simulink model "FSAC2021_V1"  (R2014a)
settings: Solver=FixedStepDiscrete  StartTime=0.0  StopTime=inf  FixedStep=0.0005  RelTol=1e-3
model workspace (MAT data in the model file):
  MCOS : class17 (value not decoded)
  MCOS : class17 (value not decoded)
  MCOS : class17 (value not decoded)
  MCOS : class17 (value not decoded)
  MCOS : class17 (value not decoded)
  MCOS : class17 (value not decoded)
  MCOS : class17 (value not decoded)
  MCOS : class17 (value not decoded)
  MCOS : class17 (value not decoded)
  MCOS : class17 (value not decoded)
  MCOS : class17 (value not decoded)
  MCOS : class17 (value not decoded)
  MCOS : class17 (value not decoded)
  MCOS : class17 (value not decoded)
  MCOS : class17 (value not decoded)
  MCOS : class17 (value not decoded)
  MCOS : class17 (value not decoded)
  MCOS : class17 (value not decoded)
  MCOS : class17 (value not decoded)
  BUZZER_START = 1
  MCOS : class17 (value not decoded)
  MCOS : class17 (value not decoded)
  MCOS : class17 (value not decoded)
  MCOS : class17 (value not decoded)
  MCOS : class17 (value not decoded)
  MCOS : class17 (value not decoded)
  MCOS : class17 (value not decoded)
  MCOS : class17 (value not decoded)
  MCOS : class17 (value not decoded)
  MCOS : class17 (value not decoded)
  MCOS : class17 (value not decoded)
  MCOS : class17 (value not decoded)
  MCOS : class17 (value not decoded)
  MCOS : class17 (value not decoded)
  MCOS : class17 (value not decoded)
  MCOS : class17 (value not decoded)
  MCOS : class17 (value not decoded)
  MCOS : class17 (value not decoded)
  MCOS : class17 (value not decoded)
  MCOS : class17 (value not decoded)
  MCOS : class17 (value not decoded)
  MCOS : class17 (value not decoded)
  MCOS : class17 (value not decoded)
  MCOS : class17 (value not decoded)
  MCOS : class17 (value not decoded)
  MCOS : class17 (value not decoded)
  MCOS : class17 (value not decoded)
  MCOS : class17 (value not decoded)
  MCOS : class17 (value not decoded)
  MCOS : class17 (value not decoded)
  MCOS : class17 (value not decoded)
  MCOS : class17 (value not decoded)
  MCOS : class17 (value not decoded)
  MCOS : class17 (value not decoded)
  MCOS : class17 (value not decoded)
  MCOS : class17 (value not decoded)
  MCOS : class17 (value not decoded)
  MCOS : class17 (value not decoded)
  Brake = 11
  MCOS : class17 (value not decoded)
  MCOS : class17 (value not decoded)
  MCOS : class17 (value not decoded)
  MCOS : class17 (value not decoded)
  MCOS : class17 (value not decoded)
  MCOS : class17 (value not decoded)
  MCOS : class17 (value not decoded)
  MCOS : class17 (value not decoded)
  Sensor_Acc_b = 101.85
  Sensor_Acc_k = -0.0185
  Str_Sen_Orig_Angle = -341
  MCOS : class17 (value not decoded)
  Tire_D = 0.47
  T = 0.05
libraries: simulink x189, ec55xxlib x135
(part 8 of 9)

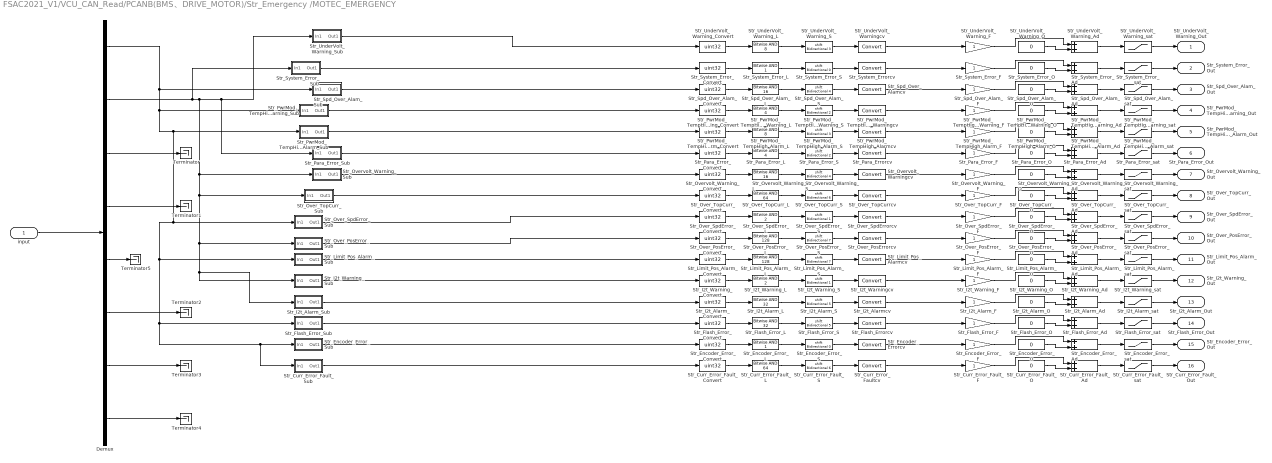
== system FSAC2021_V1/VCU_CAN_Read/PCANB(BMS、DRIVE_MOTOR)/Str_Emergency /MOTEC_EMERGENCY ==
  input : Inport
  Demux : Demux  Outputs=8
  Str_Curr_Error_Fault_Ad : Sum
  Str_Curr_Error_Fault_Convert : DataTypeConversion  OutDataTypeStr=uint32
  Str_Curr_Error_Fault_F : Gain
  Str_Curr_Error_Fault_L : simulink/Logic and Bit Operations/Bitwise Operator  logicop=AND  UseBitMask=on  BitMask=64  BitMaskRealWorld=Stored Integer
  Str_Curr_Error_Fault_O : Constant  Value=0  OutDataTypeStr=single
  Str_Curr_Error_Fault_S : ArithShift  BitShiftNumber=6
  Str_Curr_Error_Fault_Sub : Subsystem
  Str_Curr_Error_Fault_sat : Saturate  UpperLimit=1  LowerLimit=0
  Str_Curr_Error_Faultcv : DataTypeConversion
  Str_Encoder_Error_Ad : Sum
  Str_Encoder_Error_Convert : DataTypeConversion  OutDataTypeStr=uint32
  Str_Encoder_Error_F : Gain
  Str_Encoder_Error_L : simulink/Logic and Bit Operations/Bitwise Operator  logicop=AND  UseBitMask=on  BitMask=1  BitMaskRealWorld=Stored Integer
  Str_Encoder_Error_O : Constant  Value=0  OutDataTypeStr=single
  Str_Encoder_Error_S : ArithShift
  Str_Encoder_Error_Sub : Subsystem
  Str_Encoder_Error_sat : Saturate  UpperLimit=1  LowerLimit=0
  Str_Encoder_Errorcv : DataTypeConversion
  Str_Flash_Error_Ad : Sum
  Str_Flash_Error_Convert : DataTypeConversion  OutDataTypeStr=uint32
  Str_Flash_Error_F : Gain
  Str_Flash_Error_L : simulink/Logic and Bit Operations/Bitwise Operator  logicop=AND  UseBitMask=on  BitMask=32  BitMaskRealWorld=Stored Integer
  Str_Flash_Error_O : Constant  Value=0  OutDataTypeStr=single
  Str_Flash_Error_S : ArithShift  BitShiftNumber=5
  Str_Flash_Error_Sub : Subsystem
  Str_Flash_Error_sat : Saturate  UpperLimit=1  LowerLimit=0
  Str_Flash_Errorcv : DataTypeConversion
  Str_I2t_Alarm_Ad : Sum
  Str_I2t_Alarm_Convert : DataTypeConversion  OutDataTypeStr=uint32
  Str_I2t_Alarm_F : Gain
  Str_I2t_Alarm_L : simulink/Logic and Bit Operations/Bitwise Operator  logicop=AND  UseBitMask=on  BitMask=32  BitMaskRealWorld=Stored Integer
  Str_I2t_Alarm_O : Constant  Value=0  OutDataTypeStr=single
  Str_I2t_Alarm_S : ArithShift  BitShiftNumber=5
  Str_I2t_Alarm_Sub : Subsystem
  Str_I2t_Alarm_sat : Saturate  UpperLimit=1  LowerLimit=0
  Str_I2t_Alarmcv : DataTypeConversion
  Str_I2t_Warning_Ad : Sum
  Str_I2t_Warning_Convert : DataTypeConversion  OutDataTypeStr=uint32
  Str_I2t_Warning_F : Gain
  Str_I2t_Warning_L : simulink/Logic and Bit Operations/Bitwise Operator  logicop=AND  UseBitMask=on  BitMask=2  BitMaskRealWorld=Stored Integer
  Str_I2t_Warning_O : Constant  Value=0  OutDataTypeStr=single
  Str_I2t_Warning_S : ArithShift  BitShiftNumber=1
  Str_I2t_Warning_Sub : Subsystem
  Str_I2t_Warning_sat : Saturate  UpperLimit=1  LowerLimit=0
  Str_I2t_Warningcv : DataTypeConversion
  Str_Limit_Pos_Alarm_Ad : Sum
  Str_Limit_Pos_Alarm_Convert : DataTypeConversion  OutDataTypeStr=uint32
  Str_Limit_Pos_Alarm_F : Gain
  Str_Limit_Pos_Alarm_L : simulink/Logic and Bit Operations/Bitwise Operator  logicop=AND  UseBitMask=on  BitMask=128  BitMaskRealWorld=Stored Integer
  Str_Limit_Pos_Alarm_O : Constant  Value=0  OutDataTypeStr=single
  Str_Limit_Pos_Alarm_S : ArithShift  BitShiftNumber=7
  Str_Limit_Pos_Alarm_Sub : Subsystem
  Str_Limit_Pos_Alarm_sat : Saturate  UpperLimit=1  LowerLimit=0
  Str_Limit_Pos_Alarmcv : DataTypeConversion
  Str_Over_PosError_Ad : Sum
  Str_Over_PosError_Convert : DataTypeConversion  OutDataTypeStr=uint32
  Str_Over_PosError_F : Gain
  Str_Over_PosError_L : simulink/Logic and Bit Operations/Bitwise Operator  logicop=AND  UseBitMask=on  BitMask=128  BitMaskRealWorld=Stored Integer
  Str_Over_PosError_O : Constant  Value=0  OutDataTypeStr=single
  Str_Over_PosError_S : ArithShift  BitShiftNumber=7
  Str_Over_PosError_Sub : Subsystem
  Str_Over_PosError_sat : Saturate  UpperLimit=1  LowerLimit=0
  Str_Over_PosErrorcv : DataTypeConversion
  Str_Over_SpdError_Ad : Sum
  Str_Over_SpdError_Convert : DataTypeConversion  OutDataTypeStr=uint32
  Str_Over_SpdError_F : Gain
  Str_Over_SpdError_L : simulink/Logic and Bit Operations/Bitwise Operator  logicop=AND  UseBitMask=on  BitMask=2  BitMaskRealWorld=Stored Integer
  Str_Over_SpdError_O : Constant  Value=0  OutDataTypeStr=single
  Str_Over_SpdError_S : ArithShift  BitShiftNumber=1
  Str_Over_SpdError_Sub : Subsystem
  Str_Over_SpdError_sat : Saturate  UpperLimit=1  LowerLimit=0
  Str_Over_SpdErrorcv : DataTypeConversion
  Str_Over_TopCurr_Ad : Sum
  Str_Over_TopCurr_Convert : DataTypeConversion  OutDataTypeStr=uint32
  Str_Over_TopCurr_F : Gain
  Str_Over_TopCurr_L : simulink/Logic and Bit Operations/Bitwise Operator  logicop=AND  UseBitMask=on  BitMask=64  BitMaskRealWorld=Stored Integer
  Str_Over_TopCurr_O : Constant  Value=0  OutDataTypeStr=single
  Str_Over_TopCurr_S : ArithShift  BitShiftNumber=6
  Str_Over_TopCurr_Sub : Subsystem
  Str_Over_TopCurr_sat : Saturate  UpperLimit=1  LowerLimit=0
  Str_Over_TopCurrcv : DataTypeConversion
  Str_Overvolt_Warning_Ad : Sum
  Str_Overvolt_Warning_Convert : DataTypeConversion  OutDataTypeStr=uint32
  Str_Overvolt_Warning_F : Gain
  Str_Overvolt_Warning_L : simulink/Logic and Bit Operations/Bitwise Operator  logicop=AND  UseBitMask=on  BitMask=16  BitMaskRealWorld=Stored Integer
  Str_Overvolt_Warning_O : Constant  Value=0  OutDataTypeStr=single
  Str_Overvolt_Warning_S : ArithShift  BitShiftNumber=4
  Str_Overvolt_Warning_Sub : Subsystem
  Str_Overvolt_Warning_sat : Saturate  UpperLimit=1  LowerLimit=0
  Str_Overvolt_Warningcv : DataTypeConversion
  Str_Para_Error_Ad : Sum
  Str_Para_Error_Convert : DataTypeConversion  OutDataTypeStr=uint32
  Str_Para_Error_F : Gain
  Str_Para_Error_L : simulink/Logic and Bit Operations/Bitwise Operator  logicop=AND  UseBitMask=on  BitMask=4  BitMaskRealWorld=Stored Integer
  Str_Para_Error_O : Constant  Value=0  OutDataTypeStr=single
  Str_Para_Error_S : ArithShift  BitShiftNumber=2
  Str_Para_Error_Sub : Subsystem
  Str_Para_Error_sat : Saturate  UpperLimit=1  LowerLimit=0
  Str_Para_Errorcv : DataTypeConversion
  Str_PwrMod_TempHigh_Alarm_Ad : Sum
  Str_PwrMod_TempHigh_Alarm_Convert : DataTypeConversion  OutDataTypeStr=uint32
  Str_PwrMod_TempHigh_Alarm_F : Gain
  Str_PwrMod_TempHigh_Alarm_L : simulink/Logic and Bit Operations/Bitwise Operator  logicop=AND  UseBitMask=on  BitMask=8  BitMaskRealWorld=Stored Integer
  Str_PwrMod_TempHigh_Alarm_O : Constant  Value=0  OutDataTypeStr=single
  Str_PwrMod_TempHigh_Alarm_S : ArithShift  BitShiftNumber=3
  Str_PwrMod_TempHigh_Alarm_Sub : Subsystem
  Str_PwrMod_TempHigh_Alarm_sat : Saturate  UpperLimit=1  LowerLimit=0
  Str_PwrMod_TempHigh_Alarmcv : DataTypeConversion
  Str_PwrMod_TempHigh_Warning_Ad : Sum
  Str_PwrMod_TempHigh_Warning_Convert : DataTypeConversion  OutDataTypeStr=uint32
  Str_PwrMod_TempHigh_Warning_F : Gain
  Str_PwrMod_TempHigh_Warning_L : simulink/Logic and Bit Operations/Bitwise Operator  logicop=AND  UseBitMask=on  BitMask=4  BitMaskRealWorld=Stored Integer
  Str_PwrMod_TempHigh_Warning_O : Constant  Value=0  OutDataTypeStr=single
  Str_PwrMod_TempHigh_Warning_S : ArithShift  BitShiftNumber=2
  Str_PwrMod_TempHigh_Warning_Sub : Subsystem
  Str_PwrMod_TempHigh_Warning_sat : Saturate  UpperLimit=1  LowerLimit=0
  Str_PwrMod_TempHigh_Warningcv : DataTypeConversion
  Str_Spd_Over_Alam_Ad : Sum
  Str_Spd_Over_Alam_Convert : DataTypeConversion  OutDataTypeStr=uint32
  Str_Spd_Over_Alam_F : Gain
  Str_Spd_Over_Alam_L : simulink/Logic and Bit Operations/Bitwise Operator  logicop=AND  UseBitMask=on  BitMask=16  BitMaskRealWorld=Stored Integer
  Str_Spd_Over_Alam_O : Constant  Value=0  OutDataTypeStr=single
  Str_Spd_Over_Alam_S : ArithShift  BitShiftNumber=4
  Str_Spd_Over_Alam_Sub : Subsystem
  Str_Spd_Over_Alam_sat : Saturate  UpperLimit=1  LowerLimit=0
  Str_Spd_Over_Alamcv : DataTypeConversion
  Str_System_Error_Ad : Sum
  Str_System_Error_Convert : DataTypeConversion  OutDataTypeStr=uint32
  Str_System_Error_F : Gain
  Str_System_Error_L : simulink/Logic and Bit Operations/Bitwise Operator  logicop=AND  UseBitMask=on  BitMask=1  BitMaskRealWorld=Stored Integer
  Str_System_Error_O : Constant  Value=0  OutDataTypeStr=single
  Str_System_Error_S : ArithShift
  Str_System_Error_Sub : Subsystem
  Str_System_Error_sat : Saturate  UpperLimit=1  LowerLimit=0
  Str_System_Errorcv : DataTypeConversion
  Str_UnderVolt_Warning_Ad : Sum
  Str_UnderVolt_Warning_Convert : DataTypeConversion  OutDataTypeStr=uint32
  Str_UnderVolt_Warning_F : Gain
  Str_UnderVolt_Warning_L : simulink/Logic and Bit Operations/Bitwise Operator  logicop=AND  UseBitMask=on  BitMask=8  BitMaskRealWorld=Stored Integer
  Str_UnderVolt_Warning_O : Constant  Value=0  OutDataTypeStr=single
  Str_UnderVolt_Warning_S : ArithShift  BitShiftNumber=3
  Str_UnderVolt_Warning_Sub : Subsystem
  Str_UnderVolt_Warning_sat : Saturate  UpperLimit=1  LowerLimit=0
  Str_UnderVolt_Warningcv : DataTypeConversion
  Terminator{,1..5} (6 alike) : Terminator
  Str_UnderVolt_Warning_Out : Outport
  Str_System_Error_Out : Outport  Port=2
  Str_Spd_Over_Alam_Out : Outport  Port=3
  Str_PwrMod_TempHigh_Warning_Out : Outport  Port=4
  Str_PwrMod_TempHigh_Alarm_Out : Outport  Port=5
  Str_Para_Error_Out : Outport  Port=6
  Str_Overvolt_Warning_Out : Outport  Port=7
  Str_Over_TopCurr_Out : Outport  Port=8
  Str_Over_SpdError_Out : Outport  Port=9
  Str_Over_PosError_Out : Outport  Port=10
  Str_Limit_Pos_Alarm_Out : Outport  Port=11
  Str_I2t_Warning_Out : Outport  Port=12
  Str_I2t_Alarm_Out : Outport  Port=13
  Str_Flash_Error_Out : Outport  Port=14
  Str_Encoder_Error_Out : Outport  Port=15
  Str_Curr_Error_Fault_Out : Outport  Port=16
  wires:
  Str_UnderVolt_Warning_F/1 -> Str_UnderVolt_Warning_Ad/1
  Str_UnderVolt_Warning_O/1 -> Str_UnderVolt_Warning_Ad/2
  Str_UnderVolt_Warning_Ad/1 -> Str_UnderVolt_Warning_sat/1
  Str_UnderVolt_Warning_sat/1 -> Str_UnderVolt_Warning_Out/1
  Demux/2 -> Str_Para_Error_Sub/1(In1), Str_UnderVolt_Warning_Sub/1(In1), Str_I2t_Warning_Sub/1(In1), Str_I2t_Alarm_Sub/1(In1), Str_Over_PosError_Sub/1(In1), Str_Over_TopCurr_Sub/1(In1), Str_Overvolt_Warning_Sub/1(In1), Str_System_Error_Sub/1(In1)
  Str_UnderVolt_Warning_Sub/1(Out1) -> Str_UnderVolt_Warning_Convert/1
  Str_UnderVolt_Warning_Convert/1 -> Str_UnderVolt_Warning_L/1
  Str_UnderVolt_Warning_L/1 -> Str_UnderVolt_Warning_S/1
  Str_UnderVolt_Warning_S/1 -> Str_UnderVolt_Warningcv/1
  Str_UnderVolt_Warningcv/1 -> Str_UnderVolt_Warning_F/1
  Str_System_Error_F/1 -> Str_System_Error_Ad/1
  Str_System_Error_O/1 -> Str_System_Error_Ad/2
  Str_System_Error_Ad/1 -> Str_System_Error_sat/1
  Str_System_Error_sat/1 -> Str_System_Error_Out/1
  Str_System_Error_Sub/1(Out1) -> Str_System_Error_Convert/1
  Str_System_Error_Convert/1 -> Str_System_Error_L/1
  Str_System_Error_L/1 -> Str_System_Error_S/1
  Str_System_Error_S/1 -> Str_System_Errorcv/1
  Str_System_Errorcv/1 -> Str_System_Error_F/1
  Str_Spd_Over_Alam_F/1 -> Str_Spd_Over_Alam_Ad/1
  Str_Spd_Over_Alam_O/1 -> Str_Spd_Over_Alam_Ad/2
  Str_Spd_Over_Alam_Ad/1 -> Str_Spd_Over_Alam_sat/1
  Str_Spd_Over_Alam_sat/1 -> Str_Spd_Over_Alam_Out/1
  Demux/1 -> Str_Encoder_Error_Sub/1(In1), Str_Curr_Error_Fault_Sub/1(In1), Str_Flash_Error_Sub/1(In1), Str_Limit_Pos_Alarm_Sub/1(In1), Str_Over_SpdError_Sub/1(In1), Str_PwrMod_TempHigh_Alarm_Sub/1(In1), Str_PwrMod_TempHigh_Warning_Sub/1(In1), Str_Spd_Over_Alam_Sub/1(In1)
  Str_Spd_Over_Alam_Sub/1(Out1) -> Str_Spd_Over_Alam_Convert/1
  Str_Spd_Over_Alam_Convert/1 -> Str_Spd_Over_Alam_L/1
  Str_Spd_Over_Alam_L/1 -> Str_Spd_Over_Alam_S/1
  Str_Spd_Over_Alam_S/1 -> Str_Spd_Over_Alamcv/1
  Str_Spd_Over_Alamcv/1 -> Str_Spd_Over_Alam_F/1
  Str_PwrMod_TempHigh_Warning_F/1 -> Str_PwrMod_TempHigh_Warning_Ad/1
  Str_PwrMod_TempHigh_Warning_O/1 -> Str_PwrMod_TempHigh_Warning_Ad/2
  Str_PwrMod_TempHigh_Warning_Ad/1 -> Str_PwrMod_TempHigh_Warning_sat/1
  Str_PwrMod_TempHigh_Warning_sat/1 -> Str_PwrMod_TempHigh_Warning_Out/1
  Str_PwrMod_TempHigh_Warning_Sub/1(Out1) -> Str_PwrMod_TempHigh_Warning_Convert/1
  Str_PwrMod_TempHigh_Warning_Convert/1 -> Str_PwrMod_TempHigh_Warning_L/1
  Str_PwrMod_TempHigh_Warning_L/1 -> Str_PwrMod_TempHigh_Warning_S/1
  Str_PwrMod_TempHigh_Warning_S/1 -> Str_PwrMod_TempHigh_Warningcv/1
  Str_PwrMod_TempHigh_Warningcv/1 -> Str_PwrMod_TempHigh_Warning_F/1
  Str_PwrMod_TempHigh_Alarm_F/1 -> Str_PwrMod_TempHigh_Alarm_Ad/1
  Str_PwrMod_TempHigh_Alarm_O/1 -> Str_PwrMod_TempHigh_Alarm_Ad/2
  Str_PwrMod_TempHigh_Alarm_Ad/1 -> Str_PwrMod_TempHigh_Alarm_sat/1
  Str_PwrMod_TempHigh_Alarm_sat/1 -> Str_PwrMod_TempHigh_Alarm_Out/1
  Str_PwrMod_TempHigh_Alarm_Sub/1(Out1) -> Str_PwrMod_TempHigh_Alarm_Convert/1
  Str_PwrMod_TempHigh_Alarm_Convert/1 -> Str_PwrMod_TempHigh_Alarm_L/1
  Str_PwrMod_TempHigh_Alarm_L/1 -> Str_PwrMod_TempHigh_Alarm_S/1
  Str_PwrMod_TempHigh_Alarm_S/1 -> Str_PwrMod_TempHigh_Alarmcv/1
  Str_PwrMod_TempHigh_Alarmcv/1 -> Str_PwrMod_TempHigh_Alarm_F/1
  Str_Para_Error_F/1 -> Str_Para_Error_Ad/1
  Str_Para_Error_O/1 -> Str_Para_Error_Ad/2
  Str_Para_Error_Ad/1 -> Str_Para_Error_sat/1
  Str_Para_Error_sat/1 -> Str_Para_Error_Out/1
  Str_Para_Error_Sub/1(Out1) -> Str_Para_Error_Convert/1
  Str_Para_Error_Convert/1 -> Str_Para_Error_L/1
  Str_Para_Error_L/1 -> Str_Para_Error_S/1
  Str_Para_Error_S/1 -> Str_Para_Errorcv/1
  Str_Para_Errorcv/1 -> Str_Para_Error_F/1
  Str_Overvolt_Warning_F/1 -> Str_Overvolt_Warning_Ad/1
  Str_Overvolt_Warning_O/1 -> Str_Overvolt_Warning_Ad/2
  Str_Overvolt_Warning_Ad/1 -> Str_Overvolt_Warning_sat/1
  Str_Overvolt_Warning_sat/1 -> Str_Overvolt_Warning_Out/1
  Str_Overvolt_Warning_Sub/1(Out1) -> Str_Overvolt_Warning_Convert/1
  Str_Overvolt_Warning_Convert/1 -> Str_Overvolt_Warning_L/1
  Str_Overvolt_Warning_L/1 -> Str_Overvolt_Warning_S/1
  Str_Overvolt_Warning_S/1 -> Str_Overvolt_Warningcv/1
  Str_Overvolt_Warningcv/1 -> Str_Overvolt_Warning_F/1
  Str_Over_TopCurr_F/1 -> Str_Over_TopCurr_Ad/1
  Str_Over_TopCurr_O/1 -> Str_Over_TopCurr_Ad/2
  Str_Over_TopCurr_Ad/1 -> Str_Over_TopCurr_sat/1
  Str_Over_TopCurr_sat/1 -> Str_Over_TopCurr_Out/1
  Str_Over_TopCurr_Sub/1(Out1) -> Str_Over_TopCurr_Convert/1
  Str_Over_TopCurr_Convert/1 -> Str_Over_TopCurr_L/1
  Str_Over_TopCurr_L/1 -> Str_Over_TopCurr_S/1
  Str_Over_TopCurr_S/1 -> Str_Over_TopCurrcv/1
  Str_Over_TopCurrcv/1 -> Str_Over_TopCurr_F/1
  Str_Over_SpdError_F/1 -> Str_Over_SpdError_Ad/1
  Str_Over_SpdError_O/1 -> Str_Over_SpdError_Ad/2
  Str_Over_SpdError_Ad/1 -> Str_Over_SpdError_sat/1
  Str_Over_SpdError_sat/1 -> Str_Over_SpdError_Out/1
  Str_Over_SpdError_Sub/1(Out1) -> Str_Over_SpdError_Convert/1
  Str_Over_SpdError_Convert/1 -> Str_Over_SpdError_L/1
  Str_Over_SpdError_L/1 -> Str_Over_SpdError_S/1
  Str_Over_SpdError_S/1 -> Str_Over_SpdErrorcv/1
  Str_Over_SpdErrorcv/1 -> Str_Over_SpdError_F/1
  Str_Over_PosError_F/1 -> Str_Over_PosError_Ad/1
  Str_Over_PosError_O/1 -> Str_Over_PosError_Ad/2
  Str_Over_PosError_Ad/1 -> Str_Over_PosError_sat/1
  Str_Over_PosError_sat/1 -> Str_Over_PosError_Out/1
  Str_Over_PosError_Sub/1(Out1) -> Str_Over_PosError_Convert/1
  Str_Over_PosError_Convert/1 -> Str_Over_PosError_L/1
  Str_Over_PosError_L/1 -> Str_Over_PosError_S/1
  Str_Over_PosError_S/1 -> Str_Over_PosErrorcv/1
  Str_Over_PosErrorcv/1 -> Str_Over_PosError_F/1
  Str_Limit_Pos_Alarm_F/1 -> Str_Limit_Pos_Alarm_Ad/1
  Str_Limit_Pos_Alarm_O/1 -> Str_Limit_Pos_Alarm_Ad/2
  Str_Limit_Pos_Alarm_Ad/1 -> Str_Limit_Pos_Alarm_sat/1
  Str_Limit_Pos_Alarm_sat/1 -> Str_Limit_Pos_Alarm_Out/1
  Str_Limit_Pos_Alarm_Sub/1(Out1) -> Str_Limit_Pos_Alarm_Convert/1
  Str_Limit_Pos_Alarm_Convert/1 -> Str_Limit_Pos_Alarm_L/1
  Str_Limit_Pos_Alarm_L/1 -> Str_Limit_Pos_Alarm_S/1
  Str_Limit_Pos_Alarm_S/1 -> Str_Limit_Pos_Alarmcv/1
  Str_Limit_Pos_Alarmcv/1 -> Str_Limit_Pos_Alarm_F/1
  Str_I2t_Warning_F/1 -> Str_I2t_Warning_Ad/1
  Str_I2t_Warning_O/1 -> Str_I2t_Warning_Ad/2
  Str_I2t_Warning_Ad/1 -> Str_I2t_Warning_sat/1
  Str_I2t_Warning_sat/1 -> Str_I2t_Warning_Out/1
  Str_I2t_Warning_Sub/1(Out1) -> Str_I2t_Warning_Convert/1
  Str_I2t_Warning_Convert/1 -> Str_I2t_Warning_L/1
  Str_I2t_Warning_L/1 -> Str_I2t_Warning_S/1
  Str_I2t_Warning_S/1 -> Str_I2t_Warningcv/1
  Str_I2t_Warningcv/1 -> Str_I2t_Warning_F/1
  Str_I2t_Alarm_F/1 -> Str_I2t_Alarm_Ad/1
  Str_I2t_Alarm_O/1 -> Str_I2t_Alarm_Ad/2
  Str_I2t_Alarm_Ad/1 -> Str_I2t_Alarm_sat/1
  Str_I2t_Alarm_sat/1 -> Str_I2t_Alarm_Out/1
  Str_I2t_Alarm_Sub/1(Out1) -> Str_I2t_Alarm_Convert/1
  Str_I2t_Alarm_Convert/1 -> Str_I2t_Alarm_L/1
  Str_I2t_Alarm_L/1 -> Str_I2t_Alarm_S/1
  Str_I2t_Alarm_S/1 -> Str_I2t_Alarmcv/1
  Str_I2t_Alarmcv/1 -> Str_I2t_Alarm_F/1
  Str_Flash_Error_F/1 -> Str_Flash_Error_Ad/1
  Str_Flash_Error_O/1 -> Str_Flash_Error_Ad/2
  Str_Flash_Error_Ad/1 -> Str_Flash_Error_sat/1
  Str_Flash_Error_sat/1 -> Str_Flash_Error_Out/1
  Str_Flash_Error_Sub/1(Out1) -> Str_Flash_Error_Convert/1
  Str_Flash_Error_Convert/1 -> Str_Flash_Error_L/1
  Str_Flash_Error_L/1 -> Str_Flash_Error_S/1
  Str_Flash_Error_S/1 -> Str_Flash_Errorcv/1
  Str_Flash_Errorcv/1 -> Str_Flash_Error_F/1
  Str_Encoder_Error_F/1 -> Str_Encoder_Error_Ad/1
  Str_Encoder_Error_O/1 -> Str_Encoder_Error_Ad/2
  Str_Encoder_Error_Ad/1 -> Str_Encoder_Error_sat/1
  Str_Encoder_Error_sat/1 -> Str_Encoder_Error_Out/1
  Str_Encoder_Error_Sub/1(Out1) -> Str_Encoder_Error_Convert/1
  Str_Encoder_Error_Convert/1 -> Str_Encoder_Error_L/1
  Str_Encoder_Error_L/1 -> Str_Encoder_Error_S/1
  Str_Encoder_Error_S/1 -> Str_Encoder_Errorcv/1
  Str_Encoder_Errorcv/1 -> Str_Encoder_Error_F/1
  Str_Curr_Error_Fault_F/1 -> Str_Curr_Error_Fault_Ad/1
  Str_Curr_Error_Fault_O/1 -> Str_Curr_Error_Fault_Ad/2
  Str_Curr_Error_Fault_Ad/1 -> Str_Curr_Error_Fault_sat/1
  Str_Curr_Error_Fault_sat/1 -> Str_Curr_Error_Fault_Out/1
  Str_Curr_Error_Fault_Sub/1(Out1) -> Str_Curr_Error_Fault_Convert/1
  Str_Curr_Error_Fault_Convert/1 -> Str_Curr_Error_Fault_L/1
  Str_Curr_Error_Fault_L/1 -> Str_Curr_Error_Fault_S/1
  Str_Curr_Error_Fault_S/1 -> Str_Curr_Error_Faultcv/1
  Str_Curr_Error_Faultcv/1 -> Str_Curr_Error_Fault_F/1
  input/1 -> Demux/1
  Demux/3 -> Terminator/1
  Demux/4 -> Terminator1/1
  Demux/6 -> Terminator2/1
  Demux/7 -> Terminator3/1
  Demux/8 -> Terminator4/1
  Demux/5 -> Terminator5/1

== system FSAC2021_V1/VCU_CAN_Read/Subsystem/BMS_HCU_INFO /BMS_HCU_INFO ==
  input : Inport
  BatAlmLv_Ad : Sum
  BatAlmLv_Convert : DataTypeConversion  OutDataTypeStr=uint32
  BatAlmLv_F : Gain
  BatAlmLv_L : simulink/Logic and Bit Operations/Bitwise Operator  logicop=AND  UseBitMask=on  BitMask=15  BitMaskRealWorld=Stored Integer
  BatAlmLv_O : Constant  Value=0  OutDataTypeStr=single
  BatAlmLv_S : ArithShift
  BatAlmLv_Sub : Subsystem
  BatAlmLv_sat : Saturate  UpperLimit=4  LowerLimit=0
  BatAlmLvcv : DataTypeConversion
  BatCurrent_Ad : Sum
  BatCurrent_Convert : DataTypeConversion  OutDataTypeStr=uint32
  BatCurrent_F : Gain  Gain=0.1
  BatCurrent_L : simulink/Logic and Bit Operations/Bitwise Operator  logicop=AND  UseBitMask=on  BitMask=65535  BitMaskRealWorld=Stored Integer
  BatCurrent_O : Constant  Value=-1000  OutDataTypeStr=single
  BatCurrent_S : ArithShift
  BatCurrent_Sub : Subsystem
  BatCurrent_sat : Saturate  UpperLimit=1000  LowerLimit=-1000
  BatCurrentcv : DataTypeConversion
  BatCurrentinput3_Ad : Sum
  BatCurrentinput3_C : Constant  Value=256
  BatCurrentinput3_P : Product
  BatLife_Ad : Sum
  BatLife_Convert : DataTypeConversion  OutDataTypeStr=uint32
  BatLife_F : Gain
  BatLife_L : simulink/Logic and Bit Operations/Bitwise Operator  logicop=AND  UseBitMask=on  BitMask=255  BitMaskRealWorld=Stored Integer
  BatLife_O : Constant  Value=0  OutDataTypeStr=single
  BatLife_S : ArithShift
  BatLife_Sub : Subsystem
  BatLife_sat : Saturate  UpperLimit=255  LowerLimit=0
  BatLifecv : DataTypeConversion
  BatSoc_Ad : Sum
  BatSoc_Convert : DataTypeConversion  OutDataTypeStr=uint32
  BatSoc_F : Gain
  BatSoc_L : simulink/Logic and Bit Operations/Bitwise Operator  logicop=AND  UseBitMask=on  BitMask=255  BitMaskRealWorld=Stored Integer
  BatSoc_O : Constant  Value=0  OutDataTypeStr=single
  BatSoc_S : ArithShift
  BatSoc_Sub : Subsystem
  BatSoc_sat : Saturate  UpperLimit=100  LowerLimit=0
  BatSoccv : DataTypeConversion
  BatSoh_Ad : Sum
  BatSoh_Convert : DataTypeConversion  OutDataTypeStr=uint32
  BatSoh_F : Gain
  BatSoh_L : simulink/Logic and Bit Operations/Bitwise Operator  logicop=AND  UseBitMask=on  BitMask=255  BitMaskRealWorld=Stored Integer
  BatSoh_O : Constant  Value=0  OutDataTypeStr=single
  BatSoh_S : ArithShift
  BatSoh_Sub : Subsystem
  BatSoh_sat : Saturate  UpperLimit=100  LowerLimit=0
  BatSohcv : DataTypeConversion
  BatState_Ad : Sum
  BatState_Convert : DataTypeConversion  OutDataTypeStr=uint32
  BatState_F : Gain
  BatState_L : simulink/Logic and Bit Operations/Bitwise Operator  logicop=AND  UseBitMask=on  BitMask=240  BitMaskRealWorld=Stored Integer
  BatState_O : Constant  Value=0  OutDataTypeStr=single
  BatState_S : ArithShift  BitShiftNumber=4
  BatState_Sub : Subsystem
  BatState_sat : Saturate  UpperLimit=7  LowerLimit=1
  BatStatecv : DataTypeConversion
  BatVoltage_Ad : Sum
  BatVoltage_Convert : DataTypeConversion  OutDataTypeStr=uint32
  BatVoltage_F : Gain  Gain=0.1
  BatVoltage_L : simulink/Logic and Bit Operations/Bitwise Operator  logicop=AND  UseBitMask=on  BitMask=65535  BitMaskRealWorld=Stored Integer
  BatVoltage_O : Constant  Value=0  OutDataTypeStr=single
  BatVoltage_S : ArithShift
  BatVoltage_Sub : Subsystem
  BatVoltage_sat : Saturate  UpperLimit=900  LowerLimit=0
  BatVoltagecv : DataTypeConversion
  BatVoltageinput1_Ad : Sum
  BatVoltageinput1_C : Constant  Value=256
  BatVoltageinput1_P : Product
  Demux : Demux  Outputs=8
  BatLife_Out : Outport
  BatAlmLv_Out : Outport  Port=2
  BatState_Out : Outport  Port=3
  BatSoh_Out : Outport  Port=4
  BatSoc_Out : Outport  Port=5
  BatCurrent_Out : Outport  Port=6
  BatVoltage_Out : Outport  Port=7
  wires:
  BatLife_F/1 -> BatLife_Ad/1
  BatLife_O/1 -> BatLife_Ad/2
  BatLife_Ad/1 -> BatLife_sat/1
  BatLife_sat/1 -> BatLife_Out/1
  Demux/8 -> BatLife_Sub/1(In1)
  BatLife_Sub/1(Out1) -> BatLife_Convert/1
  BatLife_Convert/1 -> BatLife_L/1
  BatLife_L/1 -> BatLife_S/1
  BatLife_S/1 -> BatLifecv/1
  BatLifecv/1 -> BatLife_F/1
  BatAlmLv_F/1 -> BatAlmLv_Ad/1
  BatAlmLv_O/1 -> BatAlmLv_Ad/2
  BatAlmLv_Ad/1 -> BatAlmLv_sat/1
  BatAlmLv_sat/1 -> BatAlmLv_Out/1
  Demux/7 -> BatAlmLv_Sub/1(In1), BatState_Sub/1(In1)
  BatAlmLv_Sub/1(Out1) -> BatAlmLv_Convert/1
  BatAlmLv_Convert/1 -> BatAlmLv_L/1
  BatAlmLv_L/1 -> BatAlmLv_S/1
  BatAlmLv_S/1 -> BatAlmLvcv/1
  BatAlmLvcv/1 -> BatAlmLv_F/1
  BatState_F/1 -> BatState_Ad/1
  BatState_O/1 -> BatState_Ad/2
  BatState_Ad/1 -> BatState_sat/1
  BatState_sat/1 -> BatState_Out/1
  BatState_Sub/1(Out1) -> BatState_Convert/1
  BatState_Convert/1 -> BatState_L/1
  BatState_L/1 -> BatState_S/1
  BatState_S/1 -> BatStatecv/1
  BatStatecv/1 -> BatState_F/1
  BatSoh_F/1 -> BatSoh_Ad/1
  BatSoh_O/1 -> BatSoh_Ad/2
  BatSoh_Ad/1 -> BatSoh_sat/1
  BatSoh_sat/1 -> BatSoh_Out/1
  Demux/6 -> BatSoh_Sub/1(In1)
  BatSoh_Sub/1(Out1) -> BatSoh_Convert/1
  BatSoh_Convert/1 -> BatSoh_L/1
  BatSoh_L/1 -> BatSoh_S/1
  BatSoh_S/1 -> BatSohcv/1
  BatSohcv/1 -> BatSoh_F/1
  BatSoc_F/1 -> BatSoc_Ad/1
  BatSoc_O/1 -> BatSoc_Ad/2
  BatSoc_Ad/1 -> BatSoc_sat/1
  BatSoc_sat/1 -> BatSoc_Out/1
  Demux/5 -> BatSoc_Sub/1(In1)
  BatSoc_Sub/1(Out1) -> BatSoc_Convert/1
  BatSoc_Convert/1 -> BatSoc_L/1
  BatSoc_L/1 -> BatSoc_S/1
  BatSoc_S/1 -> BatSoccv/1
  BatSoccv/1 -> BatSoc_F/1
  BatCurrent_F/1 -> BatCurrent_Ad/1
  BatCurrent_O/1 -> BatCurrent_Ad/2
  BatCurrent_Ad/1 -> BatCurrent_sat/1
  BatCurrent_sat/1 -> BatCurrent_Out/1
  Demux/3 -> BatCurrentinput3_P/1
  BatCurrentinput3_C/1 -> BatCurrentinput3_P/2
  BatCurrentinput3_P/1 -> BatCurrentinput3_Ad/1
  Demux/4 -> BatCurrentinput3_Ad/2
  BatCurrentinput3_Ad/1 -> BatCurrent_Sub/1(In1)
  BatCurrent_Sub/1(Out1) -> BatCurrent_Convert/1
  BatCurrent_Convert/1 -> BatCurrent_L/1
  BatCurrent_L/1 -> BatCurrent_S/1
  BatCurrent_S/1 -> BatCurrentcv/1
  BatCurrentcv/1 -> BatCurrent_F/1
  BatVoltage_F/1 -> BatVoltage_Ad/1
  BatVoltage_O/1 -> BatVoltage_Ad/2
  BatVoltage_Ad/1 -> BatVoltage_sat/1
  BatVoltage_sat/1 -> BatVoltage_Out/1
  Demux/1 -> BatVoltageinput1_P/1
  BatVoltageinput1_C/1 -> BatVoltageinput1_P/2
  BatVoltageinput1_P/1 -> BatVoltageinput1_Ad/1
  Demux/2 -> BatVoltageinput1_Ad/2
  BatVoltageinput1_Ad/1 -> BatVoltage_Sub/1(In1)
  BatVoltage_Sub/1(Out1) -> BatVoltage_Convert/1
  BatVoltage_Convert/1 -> BatVoltage_L/1
  BatVoltage_L/1 -> BatVoltage_S/1
  BatVoltage_S/1 -> BatVoltagecv/1
  BatVoltagecv/1 -> BatVoltage_F/1
  input/1 -> Demux/1

== system FSAC2021_V1/VCU_CAN_Read/Subsystem1/HEARTBEAT /MOTEC_HEARTBEAT ==
  input : Inport
  Demux : Demux  Outputs=1
  Heartbeat_info_Ad : Sum
  Heartbeat_info_Convert : DataTypeConversion  OutDataTypeStr=uint32
  Heartbeat_info_F : Gain
  Heartbeat_info_L : simulink/Logic and Bit Operations/Bitwise Operator  logicop=AND  UseBitMask=on  BitMask=255  BitMaskRealWorld=Stored Integer
  Heartbeat_info_O : Constant  Value=0  OutDataTypeStr=single
  Heartbeat_info_S : ArithShift
  Heartbeat_info_Sub : Subsystem
  Heartbeat_info_sat : Saturate  UpperLimit=255  LowerLimit=0
  Heartbeat_infocv : DataTypeConversion
  Heartbeat_info_Out : Outport
  wires:
  Heartbeat_info_F/1 -> Heartbeat_info_Ad/1
  Heartbeat_info_O/1 -> Heartbeat_info_Ad/2
  Heartbeat_info_Ad/1 -> Heartbeat_info_sat/1
  Heartbeat_info_sat/1 -> Heartbeat_info_Out/1
  Demux/1 -> Heartbeat_info_Sub/1(In1)
  Heartbeat_info_Sub/1(Out1) -> Heartbeat_info_Convert/1
  Heartbeat_info_Convert/1 -> Heartbeat_info_L/1
  Heartbeat_info_L/1 -> Heartbeat_info_S/1
  Heartbeat_info_S/1 -> Heartbeat_infocv/1
  Heartbeat_infocv/1 -> Heartbeat_info_F/1
  input/1 -> Demux/1

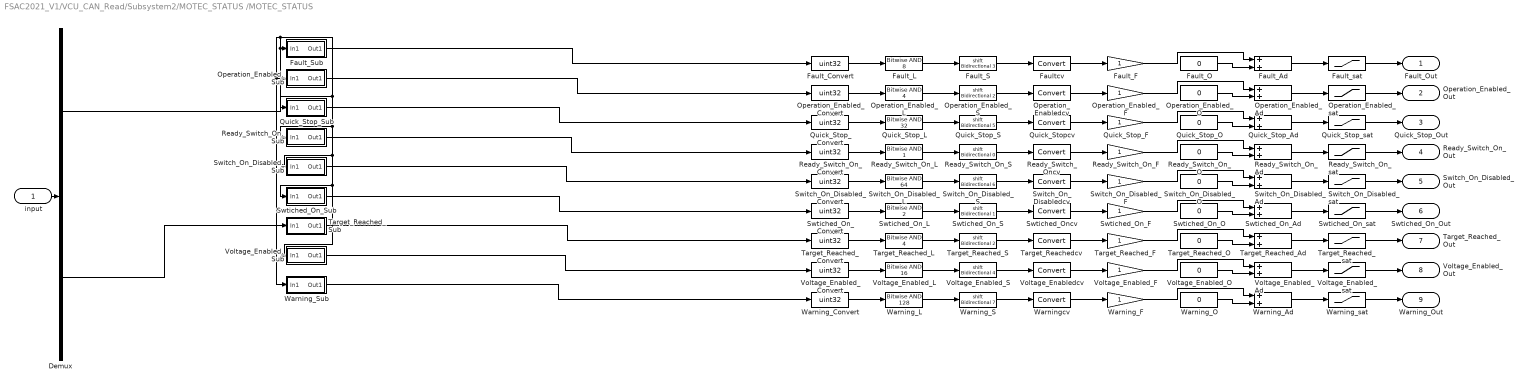
== system FSAC2021_V1/VCU_CAN_Read/Subsystem2/MOTEC_STATUS /MOTEC_STATUS ==
  input : Inport
  Demux : Demux  Outputs=2
  Fault_Ad : Sum
  Fault_Convert : DataTypeConversion  OutDataTypeStr=uint32
  Fault_F : Gain
  Fault_L : simulink/Logic and Bit Operations/Bitwise Operator  logicop=AND  UseBitMask=on  BitMask=8  BitMaskRealWorld=Stored Integer
  Fault_O : Constant  Value=0  OutDataTypeStr=single
  Fault_S : ArithShift  BitShiftNumber=3
  Fault_Sub : Subsystem
  Fault_sat : Saturate  UpperLimit=1  LowerLimit=0
  Faultcv : DataTypeConversion
  Operation_Enabled_Ad : Sum
  Operation_Enabled_Convert : DataTypeConversion  OutDataTypeStr=uint32
  Operation_Enabled_F : Gain
  Operation_Enabled_L : simulink/Logic and Bit Operations/Bitwise Operator  logicop=AND  UseBitMask=on  BitMask=4  BitMaskRealWorld=Stored Integer
  Operation_Enabled_O : Constant  Value=0  OutDataTypeStr=single
  Operation_Enabled_S : ArithShift  BitShiftNumber=2
  Operation_Enabled_Sub : Subsystem
  Operation_Enabled_sat : Saturate  UpperLimit=1  LowerLimit=0
  Operation_Enabledcv : DataTypeConversion
  Quick_Stop_Ad : Sum
  Quick_Stop_Convert : DataTypeConversion  OutDataTypeStr=uint32
  Quick_Stop_F : Gain
  Quick_Stop_L : simulink/Logic and Bit Operations/Bitwise Operator  logicop=AND  UseBitMask=on  BitMask=32  BitMaskRealWorld=Stored Integer
  Quick_Stop_O : Constant  Value=0  OutDataTypeStr=single
  Quick_Stop_S : ArithShift  BitShiftNumber=5
  Quick_Stop_Sub : Subsystem
  Quick_Stop_sat : Saturate  UpperLimit=1  LowerLimit=0
  Quick_Stopcv : DataTypeConversion
  Ready_Switch_On_Ad : Sum
  Ready_Switch_On_Convert : DataTypeConversion  OutDataTypeStr=uint32
  Ready_Switch_On_F : Gain
  Ready_Switch_On_L : simulink/Logic and Bit Operations/Bitwise Operator  logicop=AND  UseBitMask=on  BitMask=1  BitMaskRealWorld=Stored Integer
  Ready_Switch_On_O : Constant  Value=0  OutDataTypeStr=single
  Ready_Switch_On_S : ArithShift
  Ready_Switch_On_Sub : Subsystem
  Ready_Switch_On_sat : Saturate  UpperLimit=1  LowerLimit=0
  Ready_Switch_Oncv : DataTypeConversion
  Switch_On_Disabled_Ad : Sum
  Switch_On_Disabled_Convert : DataTypeConversion  OutDataTypeStr=uint32
  Switch_On_Disabled_F : Gain
  Switch_On_Disabled_L : simulink/Logic and Bit Operations/Bitwise Operator  logicop=AND  UseBitMask=on  BitMask=64  BitMaskRealWorld=Stored Integer
  Switch_On_Disabled_O : Constant  Value=0  OutDataTypeStr=single
  Switch_On_Disabled_S : ArithShift  BitShiftNumber=6
  Switch_On_Disabled_Sub : Subsystem
  Switch_On_Disabled_sat : Saturate  UpperLimit=1  LowerLimit=0
  Switch_On_Disabledcv : DataTypeConversion
  Swtiched_On_Ad : Sum
  Swtiched_On_Convert : DataTypeConversion  OutDataTypeStr=uint32
  Swtiched_On_F : Gain
  Swtiched_On_L : simulink/Logic and Bit Operations/Bitwise Operator  logicop=AND  UseBitMask=on  BitMask=2  BitMaskRealWorld=Stored Integer
  Swtiched_On_O : Constant  Value=0  OutDataTypeStr=single
  Swtiched_On_S : ArithShift  BitShiftNumber=1
  Swtiched_On_Sub : Subsystem
  Swtiched_On_sat : Saturate  UpperLimit=1  LowerLimit=0
  Swtiched_Oncv : DataTypeConversion
  Target_Reached_Ad : Sum
  Target_Reached_Convert : DataTypeConversion  OutDataTypeStr=uint32
  Target_Reached_F : Gain
  Target_Reached_L : simulink/Logic and Bit Operations/Bitwise Operator  logicop=AND  UseBitMask=on  BitMask=4  BitMaskRealWorld=Stored Integer
  Target_Reached_O : Constant  Value=0  OutDataTypeStr=single
  Target_Reached_S : ArithShift  BitShiftNumber=2
  Target_Reached_Sub : Subsystem
  Target_Reached_sat : Saturate  UpperLimit=1  LowerLimit=0
  Target_Reachedcv : DataTypeConversion
  Voltage_Enabled_Ad : Sum
  Voltage_Enabled_Convert : DataTypeConversion  OutDataTypeStr=uint32
  Voltage_Enabled_F : Gain
  Voltage_Enabled_L : simulink/Logic and Bit Operations/Bitwise Operator  logicop=AND  UseBitMask=on  BitMask=16  BitMaskRealWorld=Stored Integer
  Voltage_Enabled_O : Constant  Value=0  OutDataTypeStr=single
  Voltage_Enabled_S : ArithShift  BitShiftNumber=4
  Voltage_Enabled_Sub : Subsystem
  Voltage_Enabled_sat : Saturate  UpperLimit=1  LowerLimit=0
  Voltage_Enabledcv : DataTypeConversion
  Warning_Ad : Sum
  Warning_Convert : DataTypeConversion  OutDataTypeStr=uint32
  Warning_F : Gain
  Warning_L : simulink/Logic and Bit Operations/Bitwise Operator  logicop=AND  UseBitMask=on  BitMask=128  BitMaskRealWorld=Stored Integer
  Warning_O : Constant  Value=0  OutDataTypeStr=single
  Warning_S : ArithShift  BitShiftNumber=7
  Warning_Sub : Subsystem
  Warning_sat : Saturate  UpperLimit=1  LowerLimit=0
  Warningcv : DataTypeConversion
  Fault_Out : Outport
  Operation_Enabled_Out : Outport  Port=2
  Quick_Stop_Out : Outport  Port=3
  Ready_Switch_On_Out : Outport  Port=4
  Switch_On_Disabled_Out : Outport  Port=5
  Swtiched_On_Out : Outport  Port=6
  Target_Reached_Out : Outport  Port=7
  Voltage_Enabled_Out : Outport  Port=8
  Warning_Out : Outport  Port=9
  wires:
  Fault_F/1 -> Fault_Ad/1
  Fault_O/1 -> Fault_Ad/2
  Fault_Ad/1 -> Fault_sat/1
  Fault_sat/1 -> Fault_Out/1
  Demux/1 -> Swtiched_On_Sub/1(In1), Voltage_Enabled_Sub/1(In1), Switch_On_Disabled_Sub/1(In1), Ready_Switch_On_Sub/1(In1), Quick_Stop_Sub/1(In1), Operation_Enabled_Sub/1(In1), Warning_Sub/1(In1), Fault_Sub/1(In1)
  Fault_Sub/1(Out1) -> Fault_Convert/1
  Fault_Convert/1 -> Fault_L/1
  Fault_L/1 -> Fault_S/1
  Fault_S/1 -> Faultcv/1
  Faultcv/1 -> Fault_F/1
  Operation_Enabled_F/1 -> Operation_Enabled_Ad/1
  Operation_Enabled_O/1 -> Operation_Enabled_Ad/2
  Operation_Enabled_Ad/1 -> Operation_Enabled_sat/1
  Operation_Enabled_sat/1 -> Operation_Enabled_Out/1
  Operation_Enabled_Sub/1(Out1) -> Operation_Enabled_Convert/1
  Operation_Enabled_Convert/1 -> Operation_Enabled_L/1
  Operation_Enabled_L/1 -> Operation_Enabled_S/1
  Operation_Enabled_S/1 -> Operation_Enabledcv/1
  Operation_Enabledcv/1 -> Operation_Enabled_F/1
  Quick_Stop_F/1 -> Quick_Stop_Ad/1
  Quick_Stop_O/1 -> Quick_Stop_Ad/2
  Quick_Stop_Ad/1 -> Quick_Stop_sat/1
  Quick_Stop_sat/1 -> Quick_Stop_Out/1
  Quick_Stop_Sub/1(Out1) -> Quick_Stop_Convert/1
  Quick_Stop_Convert/1 -> Quick_Stop_L/1
  Quick_Stop_L/1 -> Quick_Stop_S/1
  Quick_Stop_S/1 -> Quick_Stopcv/1
  Quick_Stopcv/1 -> Quick_Stop_F/1
  Ready_Switch_On_F/1 -> Ready_Switch_On_Ad/1
  Ready_Switch_On_O/1 -> Ready_Switch_On_Ad/2
  Ready_Switch_On_Ad/1 -> Ready_Switch_On_sat/1
  Ready_Switch_On_sat/1 -> Ready_Switch_On_Out/1
  Ready_Switch_On_Sub/1(Out1) -> Ready_Switch_On_Convert/1
  Ready_Switch_On_Convert/1 -> Ready_Switch_On_L/1
  Ready_Switch_On_L/1 -> Ready_Switch_On_S/1
  Ready_Switch_On_S/1 -> Ready_Switch_Oncv/1
  Ready_Switch_Oncv/1 -> Ready_Switch_On_F/1
  Switch_On_Disabled_F/1 -> Switch_On_Disabled_Ad/1
  Switch_On_Disabled_O/1 -> Switch_On_Disabled_Ad/2
  Switch_On_Disabled_Ad/1 -> Switch_On_Disabled_sat/1
  Switch_On_Disabled_sat/1 -> Switch_On_Disabled_Out/1
  Switch_On_Disabled_Sub/1(Out1) -> Switch_On_Disabled_Convert/1
  Switch_On_Disabled_Convert/1 -> Switch_On_Disabled_L/1
  Switch_On_Disabled_L/1 -> Switch_On_Disabled_S/1
  Switch_On_Disabled_S/1 -> Switch_On_Disabledcv/1
  Switch_On_Disabledcv/1 -> Switch_On_Disabled_F/1
  Swtiched_On_F/1 -> Swtiched_On_Ad/1
  Swtiched_On_O/1 -> Swtiched_On_Ad/2
  Swtiched_On_Ad/1 -> Swtiched_On_sat/1
  Swtiched_On_sat/1 -> Swtiched_On_Out/1
  Swtiched_On_Sub/1(Out1) -> Swtiched_On_Convert/1
  Swtiched_On_Convert/1 -> Swtiched_On_L/1
  Swtiched_On_L/1 -> Swtiched_On_S/1
  Swtiched_On_S/1 -> Swtiched_Oncv/1
  Swtiched_Oncv/1 -> Swtiched_On_F/1
  Target_Reached_F/1 -> Target_Reached_Ad/1
  Target_Reached_O/1 -> Target_Reached_Ad/2
  Target_Reached_Ad/1 -> Target_Reached_sat/1
  Target_Reached_sat/1 -> Target_Reached_Out/1
  Demux/2 -> Target_Reached_Sub/1(In1)
  Target_Reached_Sub/1(Out1) -> Target_Reached_Convert/1
  Target_Reached_Convert/1 -> Target_Reached_L/1
  Target_Reached_L/1 -> Target_Reached_S/1
  Target_Reached_S/1 -> Target_Reachedcv/1
  Target_Reachedcv/1 -> Target_Reached_F/1
  Voltage_Enabled_F/1 -> Voltage_Enabled_Ad/1
  Voltage_Enabled_O/1 -> Voltage_Enabled_Ad/2
  Voltage_Enabled_Ad/1 -> Voltage_Enabled_sat/1
  Voltage_Enabled_sat/1 -> Voltage_Enabled_Out/1
  Voltage_Enabled_Sub/1(Out1) -> Voltage_Enabled_Convert/1
  Voltage_Enabled_Convert/1 -> Voltage_Enabled_L/1
  Voltage_Enabled_L/1 -> Voltage_Enabled_S/1
  Voltage_Enabled_S/1 -> Voltage_Enabledcv/1
  Voltage_Enabledcv/1 -> Voltage_Enabled_F/1
  Warning_F/1 -> Warning_Ad/1
  Warning_O/1 -> Warning_Ad/2
  Warning_Ad/1 -> Warning_sat/1
  Warning_sat/1 -> Warning_Out/1
  Warning_Sub/1(Out1) -> Warning_Convert/1
  Warning_Convert/1 -> Warning_L/1
  Warning_L/1 -> Warning_S/1
  Warning_S/1 -> Warningcv/1
  Warningcv/1 -> Warning_F/1
  input/1 -> Demux/1

== system FSAC2021_V1/Controller/BCU_Controller/Brk_Move/Enabled Subsystem/Angle2Pulses ==
  Angle : Inport
  Angle2Circle : Gain  Gain=-0.0028  OutDataTypeStr=single
  CircleTrans : Gain  Gain=BRK_MTR_RATIO  ParamDataTypeStr=double  OutDataTypeStr=double
  Data Type Conversion : DataTypeConversion  OutDataTypeStr=int16
  Gain : Gain  Gain=PULSES_PER_CIRCLE  ParamDataTypeStr=double  OutDataTypeStr=double
  Pulses : Outport
  wires:
  Gain/1 -> Data Type Conversion/1
  Angle2Circle/1 -> CircleTrans/1
  CircleTrans/1 -> Gain/1
  Angle/1 -> Angle2Circle/1
  Data Type Conversion/1 -> Pulses/1

== system FSAC2021_V1/Controller/BCU_Controller/Brk_Move/Enabled Subsystem1/Angle2Pulses ==
  Angle : Inport
  Angle2Circle : Gain  Gain=0.0028  OutDataTypeStr=single
  CircleTrans : Gain  Gain=BRK_MTR_RATIO  ParamDataTypeStr=double  OutDataTypeStr=double
  Data Type Conversion : DataTypeConversion  OutDataTypeStr=int16
  Gain : Gain  Gain=PULSES_PER_CIRCLE  ParamDataTypeStr=double  OutDataTypeStr=double
  Pulses : Outport
  wires:
  Gain/1 -> Data Type Conversion/1
  Angle2Circle/1 -> CircleTrans/1
  CircleTrans/1 -> Gain/1
  Angle/1 -> Angle2Circle/1
  Data Type Conversion/1 -> Pulses/1

== system FSAC2021_V1/Controller/BCU_Controller/Brk_Move/Enabled Subsystem2/Angle2Pulses ==
  Angle : Inport
  Angle2Circle : Gain  Gain=0.0028  OutDataTypeStr=single
  CircleTrans : Gain  Gain=BRK_MTR_RATIO  ParamDataTypeStr=double  OutDataTypeStr=double
  Data Type Conversion : DataTypeConversion  OutDataTypeStr=int16
  Gain : Gain  Gain=PULSES_PER_CIRCLE  ParamDataTypeStr=double  OutDataTypeStr=double
  Pulses : Outport
  wires:
  Gain/1 -> Data Type Conversion/1
  Angle2Circle/1 -> CircleTrans/1
  CircleTrans/1 -> Gain/1
  Angle/1 -> Angle2Circle/1
  Data Type Conversion/1 -> Pulses/1

== system FSAC2021_V1/Input_Process/KL_Sig_Process/Whl_Spd_Process/Whl2Veh_Spd_Trans/Round ==
  Origin_Precision : Inport
  Gain1 : Gain  Gain=10  ParamDataTypeStr=uint8  OutDataTypeStr=uint8  RndMeth=Round
  Gain2 : Gain  Gain=0.1  ParamDataTypeStr=single  OutDataTypeStr=single
  Two_Precision : Outport
  wires:
  Gain2/1 -> Two_Precision/1
  Gain1/1 -> Gain2/1
  Origin_Precision/1 -> Gain1/1

== system FSAC2021_V1/Input_Process/KL_Sig_Process/Whl_Spd_Process/Whl2Veh_Spd_Trans/Wheel_Mean ==
  Wheel_speed_rightrear_wheel : Inport
  Wheel_speed_right_front_wheel : Inport  Port=2
  Wheel_speed_leftrear_wheel : Inport  Port=3
  Wheel_speed_leftfront_wheel : Inport  Port=4
  Add3 : Sum  Inputs=++++
  Gain6 : Gain  Gain=0.25  ParamDataTypeStr=single
  Out1 : Outport
  wires:
  Wheel_speed_leftfront_wheel/1 -> Add3/4
  Wheel_speed_rightrear_wheel/1 -> Add3/1
  Wheel_speed_leftrear_wheel/1 -> Add3/3
  Wheel_speed_right_front_wheel/1 -> Add3/2
  Add3/1 -> Gain6/1
  Gain6/1 -> Out1/1

== system FSAC2021_V1/Input_Process/KL_Sig_Process/Whl_Spd_Process/Whl2Veh_Spd_Trans/rpm2km_h ==
  rpm : Inport
  Gain : Gain  Gain=2*pi*Tire_Radius*3.6/60000
  kmph : Outport
  wires:
  Gain/1 -> kmph/1
  rpm/1 -> Gain/1

== system FSAC2021_V1/VCU_CAN_Read/PCANB(BMS、DRIVE_MOTOR)/BMS_ALARM /BMS_HCU_ALARM/ALM_AUX_FAIL_Sub ==
  In1 : Inport
  Out1 : Outport
  wires:
  In1/1 -> Out1/1

== system FSAC2021_V1/VCU_CAN_Read/PCANB(BMS、DRIVE_MOTOR)/BMS_ALARM /BMS_HCU_ALARM/ALM_BATT_DT_Sub ==
  In1 : Inport
  Out1 : Outport
  wires:
  In1/1 -> Out1/1

== system FSAC2021_V1/VCU_CAN_Read/PCANB(BMS、DRIVE_MOTOR)/BMS_ALARM /BMS_HCU_ALARM/ALM_BATT_DV_Sub ==
  In1 : Inport
  Out1 : Outport
  wires:
  In1/1 -> Out1/1

== system FSAC2021_V1/VCU_CAN_Read/PCANB(BMS、DRIVE_MOTOR)/BMS_ALARM /BMS_HCU_ALARM/ALM_BATT_OC_Sub ==
  In1 : Inport
  Out1 : Outport
  wires:
  In1/1 -> Out1/1

== system FSAC2021_V1/VCU_CAN_Read/PCANB(BMS、DRIVE_MOTOR)/BMS_ALARM /BMS_HCU_ALARM/ALM_BATT_OV_Sub ==
  In1 : Inport
  Out1 : Outport
  wires:
  In1/1 -> Out1/1

== system FSAC2021_V1/VCU_CAN_Read/PCANB(BMS、DRIVE_MOTOR)/BMS_ALARM /BMS_HCU_ALARM/ALM_BATT_UC_Sub ==
  In1 : Inport
  Out1 : Outport
  wires:
  In1/1 -> Out1/1

== system FSAC2021_V1/VCU_CAN_Read/PCANB(BMS、DRIVE_MOTOR)/BMS_ALARM /BMS_HCU_ALARM/ALM_BATT_UV_Sub ==
  In1 : Inport
  Out1 : Outport
  wires:
  In1/1 -> Out1/1

== system FSAC2021_V1/VCU_CAN_Read/PCANB(BMS、DRIVE_MOTOR)/BMS_ALARM /BMS_HCU_ALARM/ALM_BMU_FAIL_Sub ==
  In1 : Inport
  Out1 : Outport
  wires:
  In1/1 -> Out1/1

== system FSAC2021_V1/VCU_CAN_Read/PCANB(BMS、DRIVE_MOTOR)/BMS_ALARM /BMS_HCU_ALARM/ALM_BSU_FAULT_Sub ==
  In1 : Inport
  Out1 : Outport
  wires:
  In1/1 -> Out1/1

== system FSAC2021_V1/VCU_CAN_Read/PCANB(BMS、DRIVE_MOTOR)/BMS_ALARM /BMS_HCU_ALARM/ALM_BSU_OFFLINE_Sub ==
  In1 : Inport
  Out1 : Outport
  wires:
  In1/1 -> Out1/1

== system FSAC2021_V1/VCU_CAN_Read/PCANB(BMS、DRIVE_MOTOR)/BMS_ALARM /BMS_HCU_ALARM/ALM_CELL_IBK_Sub ==
  In1 : Inport
  Out1 : Outport
  wires:
  In1/1 -> Out1/1

== system FSAC2021_V1/VCU_CAN_Read/PCANB(BMS、DRIVE_MOTOR)/BMS_ALARM /BMS_HCU_ALARM/ALM_CELL_OT_Sub ==
  In1 : Inport
  Out1 : Outport
  wires:
  In1/1 -> Out1/1

== system FSAC2021_V1/VCU_CAN_Read/PCANB(BMS、DRIVE_MOTOR)/BMS_ALARM /BMS_HCU_ALARM/ALM_CELL_OV_Sub ==
  In1 : Inport
  Out1 : Outport
  wires:
  In1/1 -> Out1/1

== system FSAC2021_V1/VCU_CAN_Read/PCANB(BMS、DRIVE_MOTOR)/BMS_ALARM /BMS_HCU_ALARM/ALM_CELL_TBK_Sub ==
  In1 : Inport
  Out1 : Outport
  wires:
  In1/1 -> Out1/1

== system FSAC2021_V1/VCU_CAN_Read/PCANB(BMS、DRIVE_MOTOR)/BMS_ALARM /BMS_HCU_ALARM/ALM_CELL_UT_Sub ==
  In1 : Inport
  Out1 : Outport
  wires:
  In1/1 -> Out1/1

== system FSAC2021_V1/VCU_CAN_Read/PCANB(BMS、DRIVE_MOTOR)/BMS_ALARM /BMS_HCU_ALARM/ALM_CELL_UV_Sub ==
  In1 : Inport
  Out1 : Outport
  wires:
  In1/1 -> Out1/1

== system FSAC2021_V1/VCU_CAN_Read/PCANB(BMS、DRIVE_MOTOR)/BMS_ALARM /BMS_HCU_ALARM/ALM_CHRG_OCS_Sub ==
  In1 : Inport
  Out1 : Outport
  wires:
  In1/1 -> Out1/1

== system FSAC2021_V1/VCU_CAN_Read/PCANB(BMS、DRIVE_MOTOR)/BMS_ALARM /BMS_HCU_ALARM/ALM_CHRG_OCT_Sub ==
  In1 : Inport
  Out1 : Outport
  wires:
  In1/1 -> Out1/1

== system FSAC2021_V1/VCU_CAN_Read/PCANB(BMS、DRIVE_MOTOR)/BMS_ALARM /BMS_HCU_ALARM/ALM_DSCH_OCS_Sub ==
  In1 : Inport
  Out1 : Outport
  wires:
  In1/1 -> Out1/1

== system FSAC2021_V1/VCU_CAN_Read/PCANB(BMS、DRIVE_MOTOR)/BMS_ALARM /BMS_HCU_ALARM/ALM_DSCH_OCT_Sub ==
  In1 : Inport
  Out1 : Outport
  wires:
  In1/1 -> Out1/1

== system FSAC2021_V1/VCU_CAN_Read/PCANB(BMS、DRIVE_MOTOR)/BMS_ALARM /BMS_HCU_ALARM/ALM_HALL_BREAK_Sub ==
  In1 : Inport
  Out1 : Outport
  wires:
  In1/1 -> Out1/1

== system FSAC2021_V1/VCU_CAN_Read/PCANB(BMS、DRIVE_MOTOR)/BMS_ALARM /BMS_HCU_ALARM/ALM_HVREL_FAIL_Sub ==
  In1 : Inport
  Out1 : Outport
  wires:
  In1/1 -> Out1/1

== system FSAC2021_V1/VCU_CAN_Read/PCANB(BMS、DRIVE_MOTOR)/BMS_ALARM /BMS_HCU_ALARM/ALM_LEAK_OC_Sub ==
  In1 : Inport
  Out1 : Outport
  wires:
  In1/1 -> Out1/1

== system FSAC2021_V1/VCU_CAN_Read/PCANB(BMS、DRIVE_MOTOR)/BMS_ALARM /BMS_HCU_ALARM/ALM_PRECHRG_FAIL_Sub ==
  In1 : Inport
  Out1 : Outport
  wires:
  In1/1 -> Out1/1

== system FSAC2021_V1/VCU_CAN_Read/PCANB(BMS、DRIVE_MOTOR)/BMS_ALARM /BMS_HCU_ALARM/ALM_VCU_OFFLINE_Sub ==
  In1 : Inport
  Out1 : Outport
  wires:
  In1/1 -> Out1/1

== system FSAC2021_V1/VCU_CAN_Read/PCANB(BMS、DRIVE_MOTOR)/BMS_HCU_MAXV /BMS_HCU_MAXV/MaxCellVoltNo_Sub ==
  In1 : Inport
  Out1 : Outport
  wires:
  In1/1 -> Out1/1

== system FSAC2021_V1/VCU_CAN_Read/PCANB(BMS、DRIVE_MOTOR)/BMS_HCU_MAXV /BMS_HCU_MAXV/MaxCellVolt_Sub ==
  In1 : Inport
  Out1 : Outport
  wires:
  In1/1 -> Out1/1

== system FSAC2021_V1/VCU_CAN_Read/PCANB(BMS、DRIVE_MOTOR)/BMS_HCU_MAXV /BMS_HCU_MAXV/MinCellVoltNo_Sub ==
  In1 : Inport
  Out1 : Outport
  wires:
  In1/1 -> Out1/1

== system FSAC2021_V1/VCU_CAN_Read/PCANB(BMS、DRIVE_MOTOR)/BMS_HCU_MAXV /BMS_HCU_MAXV/MinCellVolt_Sub ==
  In1 : Inport
  Out1 : Outport
  wires:
  In1/1 -> Out1/1

== system FSAC2021_V1/VCU_CAN_Read/PCANB(BMS、DRIVE_MOTOR)/BMS_HCU_POWER /BMS_HCU_POWER/MaxChrCurtLimit_Sub ==
  In1 : Inport
  Out1 : Outport
  wires:
  In1/1 -> Out1/1

== system FSAC2021_V1/VCU_CAN_Read/PCANB(BMS、DRIVE_MOTOR)/BMS_HCU_POWER /BMS_HCU_POWER/MaxChrPowerLimit_Sub ==
  In1 : Inport
  Out1 : Outport
  wires:
  In1/1 -> Out1/1

== system FSAC2021_V1/VCU_CAN_Read/PCANB(BMS、DRIVE_MOTOR)/BMS_HCU_POWER /BMS_HCU_POWER/MaxDisCurtLimit_Sub ==
  In1 : Inport
  Out1 : Outport
  wires:
  In1/1 -> Out1/1

== system FSAC2021_V1/VCU_CAN_Read/PCANB(BMS、DRIVE_MOTOR)/BMS_HCU_POWER /BMS_HCU_POWER/MaxDisPowerLimit_Sub ==
  In1 : Inport
  Out1 : Outport
  wires:
  In1/1 -> Out1/1

== system FSAC2021_V1/VCU_CAN_Read/PCANB(BMS、DRIVE_MOTOR)/BMS_RELAY /BMS_HCU_RELAY/ChrCommunication_Sub ==
  In1 : Inport
  Out1 : Outport
  wires:
  In1/1 -> Out1/1

== system FSAC2021_V1/VCU_CAN_Read/PCANB(BMS、DRIVE_MOTOR)/BMS_RELAY /BMS_HCU_RELAY/ChrReqCurr_Sub ==
  In1 : Inport
  Out1 : Outport
  wires:
  In1/1 -> Out1/1

== system FSAC2021_V1/VCU_CAN_Read/PCANB(BMS、DRIVE_MOTOR)/BMS_RELAY /BMS_HCU_RELAY/ChrReqVolt_Sub ==
  In1 : Inport
  Out1 : Outport
  wires:
  In1/1 -> Out1/1

== system FSAC2021_V1/VCU_CAN_Read/PCANB(BMS、DRIVE_MOTOR)/BMS_RELAY /BMS_HCU_RELAY/ChrState_Sub ==
  In1 : Inport
  Out1 : Outport
  wires:
  In1/1 -> Out1/1

== system FSAC2021_V1/VCU_CAN_Read/PCANB(BMS、DRIVE_MOTOR)/BMS_RELAY /BMS_HCU_RELAY/NegRlyStr_Sub ==
  In1 : Inport
  Out1 : Outport
  wires:
  In1/1 -> Out1/1

== system FSAC2021_V1/VCU_CAN_Read/PCANB(BMS、DRIVE_MOTOR)/BMS_RELAY /BMS_HCU_RELAY/OnChrRlyStr_Sub ==
  In1 : Inport
  Out1 : Outport
  wires:
  In1/1 -> Out1/1

== system FSAC2021_V1/VCU_CAN_Read/PCANB(BMS、DRIVE_MOTOR)/BMS_RELAY /BMS_HCU_RELAY/PosRlyStr_Sub ==
  In1 : Inport
  Out1 : Outport
  wires:
  In1/1 -> Out1/1

== system FSAC2021_V1/VCU_CAN_Read/PCANB(BMS、DRIVE_MOTOR)/BMS_RELAY /BMS_HCU_RELAY/PreRlyStr_Sub ==
  In1 : Inport
  Out1 : Outport
  wires:
  In1/1 -> Out1/1

== system FSAC2021_V1/VCU_CAN_Read/PCANB(BMS、DRIVE_MOTOR)/BMS_RELAY /BMS_HCU_RELAY/chrOFFCC2_Sub ==
  In1 : Inport
  Out1 : Outport
  wires:
  In1/1 -> Out1/1

== system FSAC2021_V1/VCU_CAN_Read/PCANB(BMS、DRIVE_MOTOR)/BMS_RELAY /BMS_HCU_RELAY/chrONCC_Sub ==
  In1 : Inport
  Out1 : Outport
  wires:
  In1/1 -> Out1/1

== system FSAC2021_V1/VCU_CAN_Read/PCANB(BMS、DRIVE_MOTOR)/BMS_RELAY /BMS_HCU_RELAY/offChrRlyStr_Sub ==
  In1 : Inport
  Out1 : Outport
  wires:
  In1/1 -> Out1/1

== system FSAC2021_V1/VCU_CAN_Read/PCANB(BMS、DRIVE_MOTOR)/Str_Emergency /MOTEC_EMERGENCY/Str_Curr_Error_Fault_Sub ==
  In1 : Inport
  Out1 : Outport
  wires:
  In1/1 -> Out1/1

== system FSAC2021_V1/VCU_CAN_Read/PCANB(BMS、DRIVE_MOTOR)/Str_Emergency /MOTEC_EMERGENCY/Str_Encoder_Error_Sub ==
  In1 : Inport
  Out1 : Outport
  wires:
  In1/1 -> Out1/1

== system FSAC2021_V1/VCU_CAN_Read/PCANB(BMS、DRIVE_MOTOR)/Str_Emergency /MOTEC_EMERGENCY/Str_Flash_Error_Sub ==
  In1 : Inport
  Out1 : Outport
  wires:
  In1/1 -> Out1/1

== system FSAC2021_V1/VCU_CAN_Read/PCANB(BMS、DRIVE_MOTOR)/Str_Emergency /MOTEC_EMERGENCY/Str_I2t_Alarm_Sub ==
  In1 : Inport
  Out1 : Outport
  wires:
  In1/1 -> Out1/1

== system FSAC2021_V1/VCU_CAN_Read/PCANB(BMS、DRIVE_MOTOR)/Str_Emergency /MOTEC_EMERGENCY/Str_I2t_Warning_Sub ==
  In1 : Inport
  Out1 : Outport
  wires:
  In1/1 -> Out1/1

== system FSAC2021_V1/VCU_CAN_Read/PCANB(BMS、DRIVE_MOTOR)/Str_Emergency /MOTEC_EMERGENCY/Str_Limit_Pos_Alarm_Sub ==
  In1 : Inport
  Out1 : Outport
  wires:
  In1/1 -> Out1/1

== system FSAC2021_V1/VCU_CAN_Read/PCANB(BMS、DRIVE_MOTOR)/Str_Emergency /MOTEC_EMERGENCY/Str_Over_PosError_Sub ==
  In1 : Inport
  Out1 : Outport
  wires:
  In1/1 -> Out1/1

== system FSAC2021_V1/VCU_CAN_Read/PCANB(BMS、DRIVE_MOTOR)/Str_Emergency /MOTEC_EMERGENCY/Str_Over_SpdError_Sub ==
  In1 : Inport
  Out1 : Outport
  wires:
  In1/1 -> Out1/1

== system FSAC2021_V1/VCU_CAN_Read/PCANB(BMS、DRIVE_MOTOR)/Str_Emergency /MOTEC_EMERGENCY/Str_Over_TopCurr_Sub ==
  In1 : Inport
  Out1 : Outport
  wires:
  In1/1 -> Out1/1

== system FSAC2021_V1/VCU_CAN_Read/PCANB(BMS、DRIVE_MOTOR)/Str_Emergency /MOTEC_EMERGENCY/Str_Overvolt_Warning_Sub ==
  In1 : Inport
  Out1 : Outport
  wires:
  In1/1 -> Out1/1

== system FSAC2021_V1/VCU_CAN_Read/PCANB(BMS、DRIVE_MOTOR)/Str_Emergency /MOTEC_EMERGENCY/Str_Para_Error_Sub ==
  In1 : Inport
  Out1 : Outport
  wires:
  In1/1 -> Out1/1

== system FSAC2021_V1/VCU_CAN_Read/PCANB(BMS、DRIVE_MOTOR)/Str_Emergency /MOTEC_EMERGENCY/Str_PwrMod_TempHigh_Alarm_Sub ==
  In1 : Inport
  Out1 : Outport
  wires:
  In1/1 -> Out1/1
